simulink model "q2w8"  (R2014b)
settings: Solver=ode23  StartTime=0.0  StopTime=10.0  RelTol=1e-3
undefined symbols (not defined in the file or in its folder): Kp
settings Model: Creator=Student  LastModifiedBy=Student

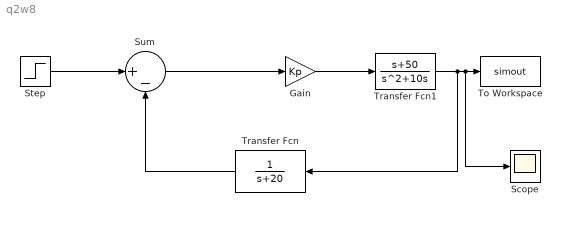
== system q2w8 ==
  Gain : Gain  Gain=Kp
  Scope : Scope
  Step : Step  SampleTime=0
  Sum : Sum  Inputs=|+-
  To Workspace : ToWorkspace  VariableName=simout  SaveFormat=Timeseries  SampleTime=-1
  Transfer Fcn : TransferFcn  Denominator=[1 20]
  Transfer Fcn1 : TransferFcn  Numerator=[1 50]  Denominator=[1 10 0]
  wires:
  Step/1 -> Sum/1
  Sum/1 -> Gain/1
  Gain/1 -> Transfer Fcn1/1
  Transfer Fcn1/1 -> Transfer Fcn/1, Scope/1, To Workspace/1
  Transfer Fcn/1 -> Sum/2
